simulink model "first_3phase"  (R2015a)
settings: Solver=ode45  StartTime=0.02  StopTime=0.06  RelTol=1e-3
libraries: powerlib x148, powerlib_meascontrol x46, simulink x34
settings Model: Creator=yahya  LastModifiedBy=Yahya

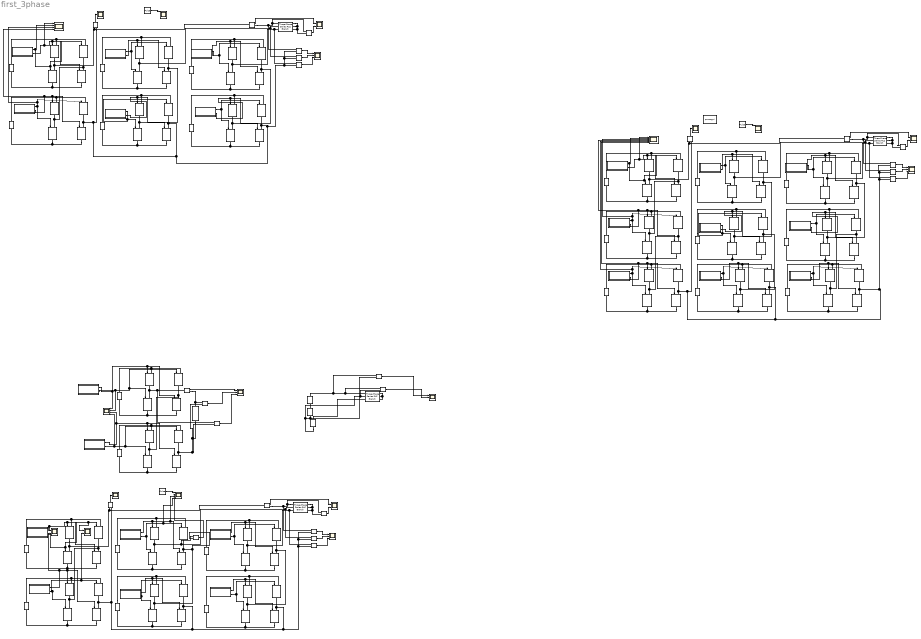
== system first_3phase ==
  note: halate adie swiching
  note: i
  note: i
  note: n
  note: i
  note: n
  note: i
  AC Voltage Source : powerlib/Electrical Sources/AC Voltage Source  Amplitude=100  Phase=0  Frequency=50  SampleTime=0  Measurements=None
  AC Voltage Source1 : powerlib/Electrical Sources/AC Voltage Source  Amplitude=100  Phase=120  Frequency=50  SampleTime=0  Measurements=None
  AC Voltage Source2 : powerlib/Electrical Sources/AC Voltage Source  Amplitude=100  Phase=120  Frequency=50  SampleTime=0  Measurements=None
  Current Measurement{1..4} (4 alike) : powerlib/Measurements/Current Measurement  PhasorSimulation=off  OutputType=Complex  PSBequivalent=0
  DC Voltage Source{1..14,18..26} (23 alike) : powerlib/Electrical Sources/DC Voltage Source  Amplitude=100  Measurements=None
  IGBT/Diode{1..56,69..104} (92 alike) : powerlib/Power Electronics/IGBT//Diode  Ron=1e-3  Rs=1e5  Cs=inf  Measurements=off
  Pulse Generator1 : DiscretePulseGenerator  PulseType=Time based  Amplitude=0.8  Period=0.0001  PulseWidth=50
  Pulse Generator2 : DiscretePulseGenerator  PulseType=Time based  Amplitude=0.8  Period=0.0002  PulseWidth=50
  Pulse Generator3 : DiscretePulseGenerator  PulseType=Time based  Amplitude=0.8  Period=0.0001  PulseWidth=50
  Scope{1,3,6,9,11} (5 alike) : Scope  NumInputPorts=4
      Scope1 settings: YMin=-5~-5~-5~-5  YMax=5~5~5~5
      Scope11 settings: YMin=-5~-5~-5~-5  YMax=5~5~5~5  SaveName=ScopeData10
      Scope3 settings: YMin=-5~-5~-5~-5  YMax=5~5~5~5  SaveName=ScopeData2
      Scope6 settings: YMin=-5~-5~-5~-5  YMax=5~5~5~5  SaveName=ScopeData12
      Scope9 settings: YMin=-5~-5~-5~-5  YMax=5~5~5~5  SaveName=ScopeData18
  Scope{2,5,10,15,17} (5 alike) : Scope  NumInputPorts=3
      Scope10 settings: YMin=-5~-5~-5  YMax=5~5~5  SaveName=ScopeData4
      Scope15 settings: TimeRange=1  YMin=-400~-400~-5  YMax=400~400~5  SaveName=ScopeData14
      Scope17 settings: YMin=-5~-5~-5  YMax=5~5~5  SaveName=ScopeData15
      Scope2 settings: YMin=-5~-5~-5  YMax=5~5~5
      Scope5 settings: TimeRange=1  YMin=-200~-200~-1  YMax=200~200~1  SaveName=ScopeData3
  Scope{4,7,12,14,18} (5 alike) : Scope  NumInputPorts=2
      Scope12 settings: TimeRange=1  YMin=-400~-400  YMax=400~400  SaveName=ScopeData5
      Scope14 settings: YMin=-5~-5  YMax=5~5  SaveName=ScopeData11
      Scope18 settings: TimeRange=1  YMin=-400~-400  YMax=400~400  SaveName=ScopeData16
      Scope4 settings: TimeRange=1  YMin=-400~-400  YMax=400~400  SaveName=ScopeData6
      Scope7 settings: YMin=-5~-5  YMax=5~5  SaveName=ScopeData13
  Scope13 : Scope
      settings: SaveName=ScopeData9
  Scope16 : Scope  NumInputPorts=6
      settings: YMin=-5~-5~-5~-5~-5~-5  YMax=5~5~5~5~5~5  SaveName=ScopeData8
  Scope19 : Scope
      settings: SaveName=ScopeData17
  Scope8 : Scope
      settings: SaveName=ScopeData7
  Series RLC Branch5 : powerlib/Elements/Series RLC Branch  LConnTagsString=__new0  RConnTagsString=__new0  BranchType=R  Resistance=1  Inductance=1e-5  SetiL0=off  InitialCurrent=0  Capacitance=1e-6  Setx0=off  InitialVoltage=0  Measurements=None
  Three-Phase Series RLC Branch : powerlib/Elements/Three-Phase Series RLC Branch  LConnTagsString=A|B|C  RConnTagsString=A|B|C  BranchType=RL  Resistance=1.405*2  Inductance=0.005839*2  Capacitance=1e-6  Measurements=Branch voltages
  Three-Phase Series RLC Branch1 : powerlib/Elements/Three-Phase Series RLC Branch  LConnTagsString=A|B|C  RConnTagsString=A|B|C  BranchType=R  Resistance=1  Inductance=1e-3  Capacitance=1e-6  Measurements=None
  Three-Phase Series RLC Branch2 : powerlib/Elements/Three-Phase Series RLC Branch  LConnTagsString=A|B|C  RConnTagsString=A|B|C  BranchType=R  Resistance=1  Inductance=1e-3  Capacitance=1e-6  Measurements=None
  Three-Phase Series RLC Branch3 : powerlib/Elements/Three-Phase Series RLC Branch  LConnTagsString=A|B|C  RConnTagsString=A|B|C  BranchType=RL  Resistance=1.405*2  Inductance=0.005839*2  Capacitance=1e-6  Measurements=Branch voltages
  Voltage Measurement{1..19} (19 alike) : powerlib/Measurements/Voltage Measurement  PhasorSimulation=off  OutputType=Complex  PSBequivalent=0
  Voltage phase n2 : powerlib/Measurements/Voltage Measurement  PhasorSimulation=off  OutputType=Complex  PSBequivalent=0
  position controller : Subsystem
  position controller1 : Subsystem
  position controller10 : Subsystem
  position controller11 : Subsystem
  position controller12 : Subsystem
  position controller13 : Subsystem
  position controller17 : Subsystem
  position controller18 : Subsystem
  position controller19 : Subsystem
  position controller2 : Subsystem
  position controller20 : Subsystem
  position controller21 : Subsystem
  position controller22 : Subsystem
  position controller23 : Subsystem
  position controller24 : Subsystem
  position controller25 : Subsystem
  position controller3 : Subsystem
  position controller4 : Subsystem
  position controller5 : Subsystem
  position controller6 : Subsystem
  position controller7 : Subsystem
  position controller8 : Subsystem
  position controller9 : Subsystem
  powergui : powerlib/powergui  Priority=1  SimulationMode=Continuous  SolverType=Tustin/Backward Euler (TBE)  SampleTime=50e-6  frequency=60  SPID=off  DisableSnubberDevices=off  DisableRonSwitches=off  DisableVfSwitches=off  SwTol=0  DisplayEquations=off  Interpol=off  methode=off  Ts=100  FunctionMessages=off  echomessages=off  HookPort=off  EnableUseOfTLC=off  x0status=blocks  frequencyindice=0  Pbase=100e6  ErrMax=1e-4  Iterations=50  UnitsV=kV  UnitsW=MW  buscounter=0  RestoreLinks=warning  ResistiveCurrentMeasurement=off  Frange=[0:2:500]  Ylog=off  Xlog=on  ShowGrid=off  save=off  variable=ZData  structure=0  ZoomFFT=on  StartTime=0.0  cycles=1  DisplayStyle=1  fundamental=60  FreqAxis=off  MaxFrequency=1000  frequencyindicesteady=1  RmsSteady=1  display=off
  wires:
  position controller/2(Out2) -> Scope11/1, IGBT/Diode35/1, IGBT/Diode21/1
  Pulse Generator1/1 -> Scope1/1
  Current Measurement2/1 -> Scope4/1
  position controller/1(Out1) -> Scope11/2, IGBT/Diode34/1, IGBT/Diode32/1
  position controller1/2(Out2) -> Scope11/4, IGBT/Diode4/1, IGBT/Diode1/1
  position controller1/1(Out1) -> IGBT/Diode3/1, Scope11/3, IGBT/Diode2/1
  position controller4/2(Out2) -> IGBT/Diode11/1, IGBT/Diode7/1
  position controller4/1(Out1) -> IGBT/Diode10/1, IGBT/Diode9/1
  position controller5/2(Out2) -> IGBT/Diode12/1, IGBT/Diode5/1
  position controller5/1(Out1) -> IGBT/Diode8/1, IGBT/Diode6/1
  position controller6/2(Out2) -> IGBT/Diode14/1, IGBT/Diode18/1
  position controller6/1(Out1) -> IGBT/Diode20/1, IGBT/Diode13/1
  position controller7/2(Out2) -> IGBT/Diode15/1, IGBT/Diode16/1
  position controller7/1(Out1) -> IGBT/Diode19/1, IGBT/Diode17/1
  position controller2/1(Out3) -> IGBT/Diode28/1, IGBT/Diode24/1, Scope3/1
  position controller2/2(Out4) -> Scope3/2, IGBT/Diode26/1, IGBT/Diode27/1
  position controller3/1(Out3) -> Scope3/3, IGBT/Diode29/1, IGBT/Diode22/1
  position controller3/2(Out4) -> Scope3/4, IGBT/Diode25/1, IGBT/Diode23/1
  Current Measurement1/1 -> Scope5/1
  Voltage Measurement5/1 -> Scope5/2
  Voltage Measurement7/1 -> Scope8/1
  Voltage Measurement4/1 -> Scope5/3
  Voltage Measurement1/1 -> Scope4/2
  Voltage Measurement2/1 -> Scope2/1
  Voltage Measurement3/1 -> Scope2/2
  Voltage Measurement6/1 -> Scope2/3
  position controller8/1(Out1) -> Scope14/1, IGBT/Diode50/1, IGBT/Diode46/1
  Current Measurement3/1 -> Scope12/1
  position controller8/2(Out2) -> IGBT/Diode49/1, Scope7/1, IGBT/Diode48/1
  position controller9/1(Out1) -> Scope14/2, IGBT/Diode51/1, IGBT/Diode30/1
  position controller9/2(Out2) -> IGBT/Diode47/1, IGBT/Diode44/1, Scope7/2
  position controller10/1(Out1) -> Scope6/3, IGBT/Diode33/1, IGBT/Diode54/1
  position controller10/2(Out2) -> Scope6/4, IGBT/Diode56/1, IGBT/Diode31/1
  position controller11/1(Out1) -> IGBT/Diode36/1, IGBT/Diode52/1
  position controller11/2(Out2) -> IGBT/Diode55/1, IGBT/Diode53/1
  position controller12/1(Out1) -> IGBT/Diode38/1, IGBT/Diode42/1
  position controller12/2(Out2) -> IGBT/Diode45/1, IGBT/Diode37/1
  position controller13/1(Out1) -> IGBT/Diode39/1, IGBT/Diode40/1
  position controller13/2(Out2) -> IGBT/Diode41/1, IGBT/Diode43/1
  Voltage phase n2/1 -> Scope13/1
  Voltage Measurement8/1 -> Scope12/2
  Voltage Measurement9/1 -> Scope10/1
  Voltage Measurement10/1 -> Scope10/2
  Voltage Measurement11/1 -> Scope10/3
  Voltage Measurement12/1 -> Scope6/2
  Pulse Generator2/1 -> Scope6/1
  Voltage Measurement14/1 -> Scope15/2
  Voltage Measurement13/1 -> Scope15/1
  position controller17/2(Out2) -> Scope16/1, IGBT/Diode86/1, IGBT/Diode82/1
  Pulse Generator3/1 -> Scope9/1
  Current Measurement4/1 -> Scope18/1
  position controller17/1(Out1) -> Scope16/2, IGBT/Diode85/1, IGBT/Diode84/1
  position controller18/2(Out2) -> Scope16/4, IGBT/Diode87/1, IGBT/Diode69/1
  position controller18/1(Out1) -> IGBT/Diode83/1, Scope16/3, IGBT/Diode80/1
  position controller22/2(Out2) -> IGBT/Diode71/1, IGBT/Diode102/1
  position controller22/1(Out1) -> IGBT/Diode70/1, IGBT/Diode104/1
  position controller23/2(Out2) -> IGBT/Diode72/1, IGBT/Diode88/1
  position controller23/1(Out1) -> IGBT/Diode103/1, IGBT/Diode92/1
  position controller24/2(Out2) -> IGBT/Diode74/1, IGBT/Diode78/1
  position controller24/1(Out1) -> IGBT/Diode81/1, IGBT/Diode73/1
  position controller25/2(Out2) -> IGBT/Diode75/1, IGBT/Diode76/1
  position controller25/1(Out1) -> IGBT/Diode79/1, IGBT/Diode77/1
  Voltage Measurement19/1 -> Scope19/1
  Voltage Measurement15/1 -> Scope18/2
  Voltage Measurement16/1 -> Scope17/1
  Voltage Measurement17/1 -> Scope17/2
  Voltage Measurement18/1 -> Scope17/3
  position controller19/2(Out2) -> Scope16/6, IGBT/Diode93/1, IGBT/Diode89/1
  position controller19/1(Out1) -> IGBT/Diode91/1, Scope16/5, IGBT/Diode90/1
  position controller20/2(Out2) -> IGBT/Diode97/1, IGBT/Diode94/1
  position controller20/1(Out1) -> IGBT/Diode96/1, IGBT/Diode95/1
  position controller21/2(Out2) -> IGBT/Diode101/1, IGBT/Diode98/1
  position controller21/1(Out1) -> IGBT/Diode100/1, IGBT/Diode99/1
  connections:
  IGBT/Diode21/LConn1 -- DC Voltage Source5/RConn1 -- IGBT/Diode32/LConn1
  IGBT/Diode35/RConn1 -- DC Voltage Source5/LConn1 -- IGBT/Diode34/RConn1
  IGBT/Diode3/LConn1 -- IGBT/Diode35/LConn1 -- IGBT/Diode32/RConn1 -- IGBT/Diode1/RConn1
  IGBT/Diode1/LConn1 -- DC Voltage Source1/RConn1 -- IGBT/Diode2/LConn1
  IGBT/Diode3/RConn1 -- DC Voltage Source1/LConn1 -- IGBT/Diode4/RConn1
  IGBT/Diode7/LConn1 -- DC Voltage Source3/RConn1 -- IGBT/Diode9/LConn1
  IGBT/Diode10/RConn1 -- DC Voltage Source3/LConn1 -- IGBT/Diode11/RConn1
  IGBT/Diode10/LConn1 -- Three-Phase Series RLC Branch/LConn2 -- Voltage Measurement3/LConn1 -- IGBT/Diode7/RConn1
  IGBT/Diode5/LConn1 -- IGBT/Diode6/LConn1 -- DC Voltage Source2/RConn1
  IGBT/Diode8/RConn1 -- DC Voltage Source2/LConn1 -- IGBT/Diode12/RConn1
  IGBT/Diode9/RConn1 -- IGBT/Diode8/LConn1 -- IGBT/Diode5/RConn1 -- IGBT/Diode11/LConn1
  IGBT/Diode18/LConn1 -- DC Voltage Source6/RConn1 -- IGBT/Diode20/LConn1
  IGBT/Diode13/RConn1 -- DC Voltage Source6/LConn1 -- IGBT/Diode14/RConn1
  IGBT/Diode16/LConn1 -- DC Voltage Source4/RConn1 -- IGBT/Diode17/LConn1
  IGBT/Diode19/RConn1 -- DC Voltage Source4/LConn1 -- IGBT/Diode15/RConn1
  IGBT/Diode20/RConn1 -- IGBT/Diode14/LConn1 -- IGBT/Diode19/LConn1 -- IGBT/Diode16/RConn1
  IGBT/Diode13/LConn1 -- Three-Phase Series RLC Branch/LConn3 -- Voltage Measurement6/LConn1 -- IGBT/Diode18/RConn1
  IGBT/Diode26/LConn1 -- IGBT/Diode24/LConn1 -- DC Voltage Source8/RConn1
  IGBT/Diode27/RConn1 -- IGBT/Diode28/RConn1 -- DC Voltage Source8/LConn1
  IGBT/Diode27/LConn1 -- Current Measurement1/LConn1 -- Voltage Measurement4/LConn1 -- IGBT/Diode24/RConn1
  IGBT/Diode23/LConn1 -- IGBT/Diode22/LConn1 -- DC Voltage Source7/RConn1
  IGBT/Diode29/RConn1 -- IGBT/Diode25/RConn1 -- DC Voltage Source7/LConn1
  IGBT/Diode28/LConn1 -- IGBT/Diode26/RConn1 -- IGBT/Diode25/LConn1 -- IGBT/Diode22/RConn1
  Series RLC Branch5/LConn1 -- Current Measurement1/RConn1 -- Voltage Measurement5/LConn1
  IGBT/Diode34/LConn1 -- IGBT/Diode21/RConn1 -- Voltage Measurement7/LConn1 -- Current Measurement2/LConn1
  Current Measurement2/RConn1 -- Voltage Measurement1/LConn1 -- Three-Phase Series RLC Branch/LConn1 -- Voltage Measurement2/LConn1
  Voltage Measurement1/LConn2 -- Three-Phase Series RLC Branch/RConn2 -- Three-Phase Series RLC Branch/RConn1 -- Three-Phase Series RLC Branch/RConn3
  IGBT/Diode48/LConn1 -- IGBT/Diode46/LConn1 -- DC Voltage Source13/RConn1
  IGBT/Diode49/RConn1 -- IGBT/Diode50/RConn1 -- DC Voltage Source13/LConn1
  IGBT/Diode30/RConn1 -- IGBT/Diode47/LConn1 -- IGBT/Diode50/LConn1 -- IGBT/Diode48/RConn1
  IGBT/Diode44/LConn1 -- IGBT/Diode30/LConn1 -- DC Voltage Source9/RConn1
  IGBT/Diode51/RConn1 -- IGBT/Diode47/RConn1 -- DC Voltage Source9/LConn1
  IGBT/Diode56/LConn1 -- IGBT/Diode54/LConn1 -- DC Voltage Source11/RConn1
  IGBT/Diode33/RConn1 -- IGBT/Diode31/RConn1 -- DC Voltage Source11/LConn1
  IGBT/Diode54/RConn1 -- Three-Phase Series RLC Branch1/LConn2 -- Voltage Measurement10/LConn1 -- Voltage Measurement12/LConn1 -- IGBT/Diode31/LConn1
  DC Voltage Source10/RConn1 -- IGBT/Diode52/LConn1 -- IGBT/Diode53/LConn1
  IGBT/Diode36/RConn1 -- IGBT/Diode55/RConn1 -- DC Voltage Source10/LConn1
  IGBT/Diode33/LConn1 -- IGBT/Diode56/RConn1 -- IGBT/Diode55/LConn1 -- IGBT/Diode52/RConn1 -- Voltage Measurement12/LConn2
  IGBT/Diode45/LConn1 -- DC Voltage Source14/RConn1 -- IGBT/Diode42/LConn1
  IGBT/Diode38/RConn1 -- IGBT/Diode37/RConn1 -- DC Voltage Source14/LConn1
  IGBT/Diode41/LConn1 -- DC Voltage Source12/RConn1 -- IGBT/Diode40/LConn1
  IGBT/Diode39/RConn1 -- IGBT/Diode43/RConn1 -- DC Voltage Source12/LConn1
  IGBT/Diode40/RConn1 -- IGBT/Diode43/LConn1 -- IGBT/Diode45/RConn1 -- IGBT/Diode38/LConn1
  IGBT/Diode42/RConn1 -- Three-Phase Series RLC Branch1/LConn3 -- Voltage Measurement11/LConn1 -- IGBT/Diode37/LConn1
  Voltage phase n2/LConn1 -- Current Measurement3/LConn1 -- IGBT/Diode49/LConn1 -- IGBT/Diode46/RConn1
  Three-Phase Series RLC Branch1/LConn1 -- Voltage Measurement9/LConn1 -- Current Measurement3/RConn1 -- Voltage Measurement8/LConn1
  Three-Phase Series RLC Branch1/RConn1 -- Voltage Measurement8/LConn2 -- Three-Phase Series RLC Branch1/RConn3 -- Three-Phase Series RLC Branch1/RConn2
  IGBT/Diode53/RConn1 -- IGBT/Diode39/LConn1 -- IGBT/Diode41/RConn1 -- Voltage Measurement11/LConn2 -- Voltage Measurement9/LConn2 -- Voltage Measurement10/LConn2 -- Voltage phase n2/LConn2 -- IGBT/Diode51/LConn1 -- IGBT/Diode44/RConn1 -- IGBT/Diode36/LConn1
  AC Voltage Source1/LConn1 -- AC Voltage Source/LConn1 -- AC Voltage Source2/LConn1 -- Voltage Measurement13/LConn2
  AC Voltage Source/RConn1 -- Voltage Measurement13/LConn1 -- Voltage Measurement14/LConn1 -- Three-Phase Series RLC Branch2/LConn1
  AC Voltage Source1/RConn1 -- Voltage Measurement14/LConn2 -- Three-Phase Series RLC Branch2/LConn2
  AC Voltage Source2/RConn1 -- Three-Phase Series RLC Branch2/LConn3
  Three-Phase Series RLC Branch2/RConn1 -- Three-Phase Series RLC Branch2/RConn3 -- Three-Phase Series RLC Branch2/RConn2
  Voltage Measurement5/LConn2 -- Series RLC Branch5/RConn1 -- IGBT/Diode29/LConn1 -- IGBT/Diode23/RConn1 -- Voltage Measurement4/LConn2
  IGBT/Diode4/LConn1 -- Voltage Measurement6/LConn2 -- Voltage Measurement2/LConn2 -- Voltage Measurement3/LConn2 -- IGBT/Diode17/RConn1 -- IGBT/Diode15/LConn1 -- IGBT/Diode6/RConn1 -- IGBT/Diode12/LConn1 -- Voltage Measurement7/LConn2 -- IGBT/Diode2/RConn1
  IGBT/Diode84/LConn1 -- IGBT/Diode82/LConn1 -- DC Voltage Source25/RConn1
  IGBT/Diode85/RConn1 -- IGBT/Diode86/RConn1 -- DC Voltage Source25/LConn1
  IGBT/Diode69/RConn1 -- IGBT/Diode83/LConn1 -- IGBT/Diode86/LConn1 -- IGBT/Diode84/RConn1
  IGBT/Diode80/LConn1 -- IGBT/Diode69/LConn1 -- DC Voltage Source18/RConn1
  IGBT/Diode87/RConn1 -- IGBT/Diode83/RConn1 -- DC Voltage Source18/LConn1
  IGBT/Diode104/LConn1 -- IGBT/Diode102/LConn1 -- DC Voltage Source23/RConn1
  IGBT/Diode71/RConn1 -- IGBT/Diode70/RConn1 -- DC Voltage Source23/LConn1
  IGBT/Diode102/RConn1 -- IGBT/Diode70/LConn1 -- Three-Phase Series RLC Branch3/LConn2 -- Voltage Measurement17/LConn1
  DC Voltage Source22/RConn1 -- IGBT/Diode88/LConn1 -- IGBT/Diode92/LConn1
  IGBT/Diode72/RConn1 -- IGBT/Diode103/RConn1 -- DC Voltage Source22/LConn1
  IGBT/Diode71/LConn1 -- IGBT/Diode104/RConn1 -- IGBT/Diode103/LConn1 -- IGBT/Diode88/RConn1
  IGBT/Diode81/LConn1 -- IGBT/Diode78/LConn1 -- DC Voltage Source26/RConn1
  IGBT/Diode74/RConn1 -- IGBT/Diode73/RConn1 -- DC Voltage Source26/LConn1
  IGBT/Diode77/LConn1 -- IGBT/Diode76/LConn1 -- DC Voltage Source24/RConn1
  IGBT/Diode75/RConn1 -- IGBT/Diode79/RConn1 -- DC Voltage Source24/LConn1
  IGBT/Diode76/RConn1 -- IGBT/Diode79/LConn1 -- IGBT/Diode81/RConn1 -- IGBT/Diode74/LConn1
  IGBT/Diode78/RConn1 -- Three-Phase Series RLC Branch3/LConn3 -- Voltage Measurement18/LConn1 -- IGBT/Diode73/LConn1
  Current Measurement4/LConn1 -- Voltage Measurement19/LConn1 -- IGBT/Diode85/LConn1 -- IGBT/Diode82/RConn1
  Voltage Measurement16/LConn1 -- Current Measurement4/RConn1 -- Voltage Measurement15/LConn1 -- Three-Phase Series RLC Branch3/LConn1
  Three-Phase Series RLC Branch3/RConn3 -- Voltage Measurement15/LConn2 -- Three-Phase Series RLC Branch3/RConn2 -- Three-Phase Series RLC Branch3/RConn1
  IGBT/Diode91/LConn1 -- IGBT/Diode80/RConn1 -- IGBT/Diode87/LConn1 -- IGBT/Diode89/RConn1
  IGBT/Diode96/LConn1 -- IGBT/Diode92/RConn1 -- IGBT/Diode72/LConn1 -- IGBT/Diode94/RConn1
  IGBT/Diode100/LConn1 -- IGBT/Diode77/RConn1 -- IGBT/Diode75/LConn1 -- IGBT/Diode98/RConn1
  IGBT/Diode90/LConn1 -- IGBT/Diode89/LConn1 -- DC Voltage Source19/RConn1
  IGBT/Diode93/RConn1 -- IGBT/Diode91/RConn1 -- DC Voltage Source19/LConn1
  IGBT/Diode95/LConn1 -- IGBT/Diode94/LConn1 -- DC Voltage Source20/RConn1
  IGBT/Diode97/RConn1 -- IGBT/Diode96/RConn1 -- DC Voltage Source20/LConn1
  IGBT/Diode99/LConn1 -- IGBT/Diode98/LConn1 -- DC Voltage Source21/RConn1
  IGBT/Diode101/RConn1 -- IGBT/Diode100/RConn1 -- DC Voltage Source21/LConn1
  IGBT/Diode95/RConn1 -- IGBT/Diode97/LConn1 -- Voltage Measurement16/LConn2 -- Voltage Measurement17/LConn2 -- Voltage Measurement18/LConn2 -- IGBT/Diode99/RConn1 -- IGBT/Diode101/LConn1 -- Voltage Measurement19/LConn2 -- IGBT/Diode90/RConn1 -- IGBT/Diode93/LConn1

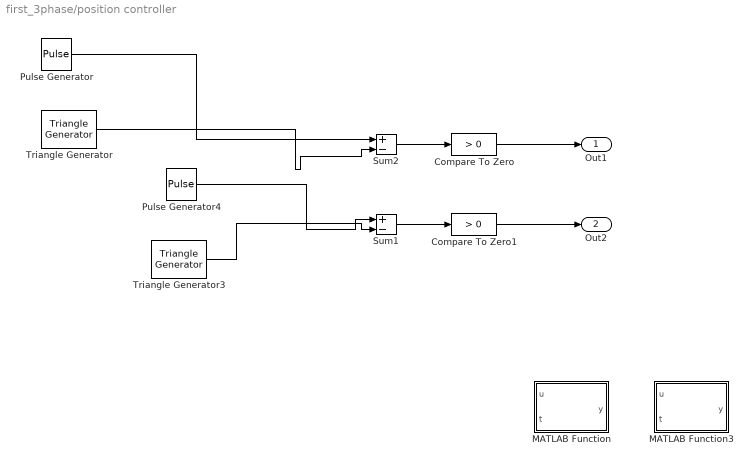
== system first_3phase/position controller ==
  Compare To Zero : simulink/Logic and Bit Operations/Compare To Zero  relop=>  OutDataTypeStr=boolean  ZeroCross=off
  Compare To Zero1 : simulink/Logic and Bit Operations/Compare To Zero  relop=>  OutDataTypeStr=boolean  ZeroCross=off
  MATLAB Function : MATLAB Function  TreatAsAtomicUnit=on
  MATLAB Function3 : MATLAB Function  TreatAsAtomicUnit=on
  Pulse Generator : DiscretePulseGenerator  PulseType=Time based  Amplitude=0.666  Period=0.02  PulseWidth=50
  Pulse Generator4 : DiscretePulseGenerator  PulseType=Time based  Amplitude=0.666  Period=0.02  PulseWidth=50  PhaseDelay=0.01
  Sum1 : Sum  Inputs=+-  OutDataTypeStr=double
  Sum2 : Sum  Inputs=+-  OutDataTypeStr=double
  Triangle Generator : powerlib_meascontrol/Pulse & Signal Generators/Triangle Generator  Freq=50  Phase=90  Ts=0
  Triangle Generator3 : powerlib_meascontrol/Pulse & Signal Generators/Triangle Generator  Freq=50  Phase=90+180  Ts=0
  Out1 : Outport
  Out2 : Outport  Port=2
  wires:
  Compare To Zero/1 -> Out1/1
  Pulse Generator/1 -> Sum2/1
  Triangle Generator/1 -> Sum2/2
  Pulse Generator4/1 -> Sum1/1
  Triangle Generator3/1 -> Sum1/2
  Compare To Zero1/1 -> Out2/1
  Sum2/1 -> Compare To Zero/1
  Sum1/1 -> Compare To Zero1/1

== system first_3phase/position controller1 ==
  Compare To Zero : simulink/Logic and Bit Operations/Compare To Zero  relop=>  OutDataTypeStr=boolean  ZeroCross=off
  Compare To Zero1 : simulink/Logic and Bit Operations/Compare To Zero  relop=>  OutDataTypeStr=boolean  ZeroCross=off
  Pulse Generator5 : DiscretePulseGenerator  PulseType=Time based  Amplitude=0.333  Period=0.02  PulseWidth=50
  Pulse Generator6 : DiscretePulseGenerator  PulseType=Time based  Amplitude=0.333  Period=0.02  PulseWidth=50  PhaseDelay=0.01
  Sum1 : Sum  Inputs=+-  OutDataTypeStr=double
  Sum2 : Sum  Inputs=+-  OutDataTypeStr=double
  Triangle Generator4 : powerlib_meascontrol/Pulse & Signal Generators/Triangle Generator  Freq=50  Phase=90  Ts=0
  Triangle Generator5 : powerlib_meascontrol/Pulse & Signal Generators/Triangle Generator  Freq=50  Phase=90+180  Ts=0
  Out1 : Outport
  Out2 : Outport  Port=2
  wires:
  Compare To Zero/1 -> Out1/1
  Compare To Zero1/1 -> Out2/1
  Pulse Generator5/1 -> Sum2/1
  Triangle Generator4/1 -> Sum2/2
  Pulse Generator6/1 -> Sum1/1
  Triangle Generator5/1 -> Sum1/2
  Sum2/1 -> Compare To Zero/1
  Sum1/1 -> Compare To Zero1/1

== system first_3phase/position controller10 ==
  Clock : Clock
  Pulse Generator7 : DiscretePulseGenerator  PulseType=Time based  Period=0.02  PulseWidth=50  PhaseDelay=0.00666
  Pulse Generator8 : DiscretePulseGenerator  PulseType=Time based  Period=0.02  PulseWidth=50  PhaseDelay=0.01+0.00666
  Triangle Generator6 : powerlib_meascontrol/Pulse & Signal Generators/Triangle Generator  Freq=50  Phase=90+240  Ts=0
  Triangle Generator7 : powerlib_meascontrol/Pulse & Signal Generators/Triangle Generator  Freq=50  Phase=90+180+240  Ts=0
  Out1 : Outport
  Out2 : Outport  Port=2
  wires:
  Pulse Generator7/1 -> Out1/1
  Pulse Generator8/1 -> Out2/1
  Triangle Generator6/1 -> ?
  Triangle Generator7/1 -> ?
  Clock/1 -> ?

== system first_3phase/position controller11 ==
  Clock : Clock
  MATLAB Function8 : MATLAB Function  TreatAsAtomicUnit=on
  MATLAB Function9 : MATLAB Function  TreatAsAtomicUnit=on
  Pulse Generator10 : DiscretePulseGenerator  PulseType=Time based  Amplitude=0.332  Period=0.02  PulseWidth=50  PhaseDelay=0.01+0.00666
  Pulse Generator9 : DiscretePulseGenerator  PulseType=Time based  Amplitude=0.332  Period=0.02  PulseWidth=50  PhaseDelay=0.00666
  Triangle Generator8 : powerlib_meascontrol/Pulse & Signal Generators/Triangle Generator  Freq=50  Phase=90+240  Ts=0
  Triangle Generator9 : powerlib_meascontrol/Pulse & Signal Generators/Triangle Generator  Freq=50  Phase=90+180+240  Ts=0
  Out1 : Outport
  Out2 : Outport  Port=2
  wires:
  MATLAB Function8/1(y) -> Out1/1
  Pulse Generator9/1 -> MATLAB Function8/1(u)
  Triangle Generator8/1 -> MATLAB Function8/2(t)
  MATLAB Function9/1(y) -> Out2/1
  Pulse Generator10/1 -> MATLAB Function9/1(u)
  Triangle Generator9/1 -> MATLAB Function9/3(t)
  Clock/1 -> MATLAB Function9/2(c)

== system first_3phase/position controller12 ==
  Clock : Clock
  Pulse Generator12 : DiscretePulseGenerator  PulseType=Time based  Period=0.02  PulseWidth=50  PhaseDelay=0.00666*2
  Pulse Generator13 : DiscretePulseGenerator  PulseType=Time based  Period=0.02  PulseWidth=50  PhaseDelay=0.01+0.00666*2
  Triangle Generator10 : powerlib_meascontrol/Pulse & Signal Generators/Triangle Generator  Freq=50  Phase=90+120  Ts=0
  Triangle Generator11 : powerlib_meascontrol/Pulse & Signal Generators/Triangle Generator  Freq=50  Phase=90+180+120  Ts=0
  Out1 : Outport
  Out2 : Outport  Port=2
  wires:
  Pulse Generator12/1 -> Out1/1
  Pulse Generator13/1 -> Out2/1
  Triangle Generator10/1 -> ?
  Triangle Generator11/1 -> ?
  Clock/1 -> ?

== system first_3phase/position controller13 ==
  Clock : Clock
  Pulse Generator11 : DiscretePulseGenerator  PulseType=Time based  Period=0.02  PulseWidth=50  PhaseDelay=0.01+0.00666*2
  Pulse Generator14 : DiscretePulseGenerator  PulseType=Time based  Amplitude=2  Period=0.02  PulseWidth=50  PhaseDelay=0.00666*2
  Triangle Generator12 : powerlib_meascontrol/Pulse & Signal Generators/Triangle Generator  Freq=50  Phase=90+120  Ts=0
  Triangle Generator13 : powerlib_meascontrol/Pulse & Signal Generators/Triangle Generator  Freq=50  Phase=90+180+120  Ts=0
  Out1 : Outport
  Out2 : Outport  Port=2
  wires:
  Pulse Generator14/1 -> Out1/1
  Pulse Generator11/1 -> Out2/1
  Triangle Generator12/1 -> ?
  Triangle Generator13/1 -> ?
  Clock/1 -> ?

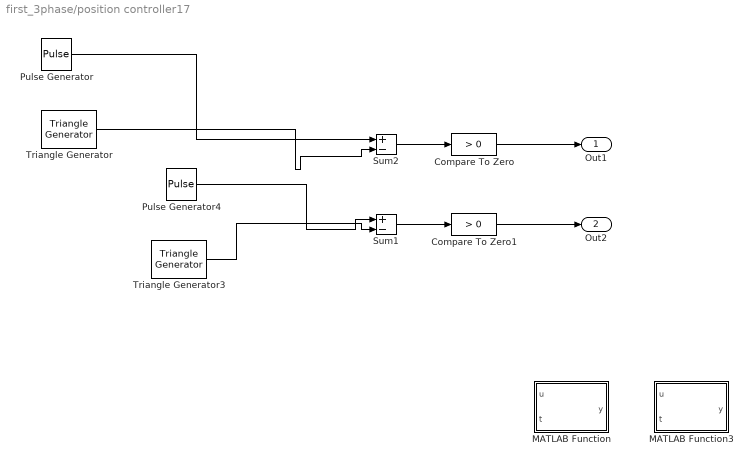
== system first_3phase/position controller17 ==
  Compare To Zero : simulink/Logic and Bit Operations/Compare To Zero  relop=>  OutDataTypeStr=boolean  ZeroCross=off
  Compare To Zero1 : simulink/Logic and Bit Operations/Compare To Zero  relop=>  OutDataTypeStr=boolean  ZeroCross=off
  MATLAB Function : MATLAB Function  TreatAsAtomicUnit=on
  MATLAB Function3 : MATLAB Function  TreatAsAtomicUnit=on
  Pulse Generator : DiscretePulseGenerator  PulseType=Time based  Amplitude=0.9774  Period=0.02  PulseWidth=50
  Pulse Generator4 : DiscretePulseGenerator  PulseType=Time based  Amplitude=0.9774  Period=0.02  PulseWidth=50  PhaseDelay=0.01
  Sum1 : Sum  Inputs=+-  OutDataTypeStr=double
  Sum2 : Sum  Inputs=+-  OutDataTypeStr=double
  Triangle Generator : powerlib_meascontrol/Pulse & Signal Generators/Triangle Generator  Freq=50  Phase=90  Ts=0
  Triangle Generator3 : powerlib_meascontrol/Pulse & Signal Generators/Triangle Generator  Freq=50  Phase=90+180  Ts=0
  Out1 : Outport
  Out2 : Outport  Port=2
  wires:
  Compare To Zero/1 -> Out1/1
  Pulse Generator/1 -> Sum2/1
  Triangle Generator/1 -> Sum2/2
  Pulse Generator4/1 -> Sum1/1
  Triangle Generator3/1 -> Sum1/2
  Compare To Zero1/1 -> Out2/1
  Sum2/1 -> Compare To Zero/1
  Sum1/1 -> Compare To Zero1/1

== system first_3phase/position controller18 ==
  Compare To Zero : simulink/Logic and Bit Operations/Compare To Zero  relop=>  OutDataTypeStr=boolean  ZeroCross=off
  Compare To Zero1 : simulink/Logic and Bit Operations/Compare To Zero  relop=>  OutDataTypeStr=boolean  ZeroCross=off
  Pulse Generator5 : DiscretePulseGenerator  PulseType=Time based  Amplitude=0.9502  Period=0.02  PulseWidth=50
  Pulse Generator6 : DiscretePulseGenerator  PulseType=Time based  Amplitude=0.9502  Period=0.02  PulseWidth=50  PhaseDelay=0.01
  Sum1 : Sum  Inputs=+-  OutDataTypeStr=double
  Sum2 : Sum  Inputs=+-  OutDataTypeStr=double
  Triangle Generator4 : powerlib_meascontrol/Pulse & Signal Generators/Triangle Generator  Freq=50  Phase=90  Ts=0
  Triangle Generator5 : powerlib_meascontrol/Pulse & Signal Generators/Triangle Generator  Freq=50  Phase=90+180  Ts=0
  Out1 : Outport
  Out2 : Outport  Port=2
  wires:
  Compare To Zero/1 -> Out1/1
  Compare To Zero1/1 -> Out2/1
  Pulse Generator5/1 -> Sum2/1
  Triangle Generator4/1 -> Sum2/2
  Pulse Generator6/1 -> Sum1/1
  Triangle Generator5/1 -> Sum1/2
  Sum2/1 -> Compare To Zero/1
  Sum1/1 -> Compare To Zero1/1

== system first_3phase/position controller19 ==
  Compare To Zero : simulink/Logic and Bit Operations/Compare To Zero  relop=>  OutDataTypeStr=boolean  ZeroCross=off
  Compare To Zero1 : simulink/Logic and Bit Operations/Compare To Zero  relop=>  OutDataTypeStr=boolean  ZeroCross=off
  Pulse Generator5 : DiscretePulseGenerator  PulseType=Time based  Amplitude=0.5294  Period=0.02  PulseWidth=50
  Pulse Generator6 : DiscretePulseGenerator  PulseType=Time based  Amplitude=0.5294  Period=0.02  PulseWidth=50  PhaseDelay=0.01
  Sum1 : Sum  Inputs=+-  OutDataTypeStr=double
  Sum2 : Sum  Inputs=+-  OutDataTypeStr=double
  Triangle Generator4 : powerlib_meascontrol/Pulse & Signal Generators/Triangle Generator  Freq=50  Phase=90  Ts=0
  Triangle Generator5 : powerlib_meascontrol/Pulse & Signal Generators/Triangle Generator  Freq=50  Phase=90+180  Ts=0
  Out1 : Outport
  Out2 : Outport  Port=2
  wires:
  Compare To Zero/1 -> Out1/1
  Compare To Zero1/1 -> Out2/1
  Pulse Generator5/1 -> Sum2/1
  Triangle Generator4/1 -> Sum2/2
  Pulse Generator6/1 -> Sum1/1
  Triangle Generator5/1 -> Sum1/2
  Sum2/1 -> Compare To Zero/1
  Sum1/1 -> Compare To Zero1/1

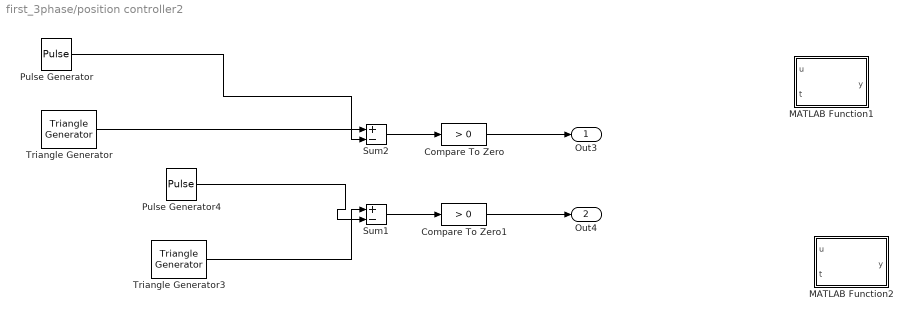
== system first_3phase/position controller2 ==
  Compare To Zero : simulink/Logic and Bit Operations/Compare To Zero  relop=>  OutDataTypeStr=boolean  ZeroCross=off
  Compare To Zero1 : simulink/Logic and Bit Operations/Compare To Zero  relop=>  OutDataTypeStr=boolean  ZeroCross=off
  MATLAB Function1 : MATLAB Function  TreatAsAtomicUnit=on
  MATLAB Function2 : MATLAB Function  TreatAsAtomicUnit=on
  Pulse Generator : DiscretePulseGenerator  PulseType=Time based  Amplitude=0.666  Period=0.02  PulseWidth=50.001
  Pulse Generator4 : DiscretePulseGenerator  PulseType=Time based  Amplitude=0.666  Period=0.02  PulseWidth=50.001  PhaseDelay=0.01
  Sum1 : Sum  Inputs=+-  OutDataTypeStr=double
  Sum2 : Sum  Inputs=+-  OutDataTypeStr=double
  Triangle Generator : powerlib_meascontrol/Pulse & Signal Generators/Triangle Generator  Freq=50  Phase=90  Ts=0
  Triangle Generator3 : powerlib_meascontrol/Pulse & Signal Generators/Triangle Generator  Freq=50  Phase=90+180  Ts=0
  Out3 : Outport
  Out4 : Outport  Port=2
  wires:
  Compare To Zero/1 -> Out3/1
  Pulse Generator/1 -> Sum2/2
  Triangle Generator/1 -> Sum2/1
  Pulse Generator4/1 -> Sum1/2
  Triangle Generator3/1 -> Sum1/1
  Compare To Zero1/1 -> Out4/1
  Sum2/1 -> Compare To Zero/1
  Sum1/1 -> Compare To Zero1/1

== system first_3phase/position controller20 ==
  Compare To Zero : simulink/Logic and Bit Operations/Compare To Zero  relop=>  OutDataTypeStr=boolean  ZeroCross=off
  Compare To Zero1 : simulink/Logic and Bit Operations/Compare To Zero  relop=>  OutDataTypeStr=boolean  ZeroCross=off
  Pulse Generator5 : DiscretePulseGenerator  PulseType=Time based  Amplitude=0.5294  Period=0.02  PulseWidth=50
  Pulse Generator6 : DiscretePulseGenerator  PulseType=Time based  Amplitude=0.5294  Period=0.02  PulseWidth=50  PhaseDelay=0.01
  Sum1 : Sum  Inputs=+-  OutDataTypeStr=double
  Sum2 : Sum  Inputs=+-  OutDataTypeStr=double
  Triangle Generator4 : powerlib_meascontrol/Pulse & Signal Generators/Triangle Generator  Freq=50  Phase=90+240  Ts=0
  Triangle Generator5 : powerlib_meascontrol/Pulse & Signal Generators/Triangle Generator  Freq=50  Phase=90+180+240  Ts=0
  Out1 : Outport
  Out2 : Outport  Port=2
  wires:
  Compare To Zero/1 -> Out1/1
  Compare To Zero1/1 -> Out2/1
  Pulse Generator5/1 -> Sum2/1
  Triangle Generator4/1 -> Sum2/2
  Pulse Generator6/1 -> Sum1/1
  Triangle Generator5/1 -> Sum1/2
  Sum2/1 -> Compare To Zero/1
  Sum1/1 -> Compare To Zero1/1

== system first_3phase/position controller21 ==
  Compare To Zero : simulink/Logic and Bit Operations/Compare To Zero  relop=>  OutDataTypeStr=boolean  ZeroCross=off
  Compare To Zero1 : simulink/Logic and Bit Operations/Compare To Zero  relop=>  OutDataTypeStr=boolean  ZeroCross=off
  Pulse Generator5 : DiscretePulseGenerator  PulseType=Time based  Amplitude=0.5294  Period=0.535476666666667  PulseWidth=50
  Pulse Generator6 : DiscretePulseGenerator  PulseType=Time based  Amplitude=0.5294  Period=0.02  PulseWidth=50  PhaseDelay=0.01
  Sum1 : Sum  Inputs=+-  OutDataTypeStr=double
  Sum2 : Sum  Inputs=+-  OutDataTypeStr=double
  Triangle Generator4 : powerlib_meascontrol/Pulse & Signal Generators/Triangle Generator  Freq=50  Phase=90+120  Ts=0
  Triangle Generator5 : powerlib_meascontrol/Pulse & Signal Generators/Triangle Generator  Freq=50  Phase=90+180+120  Ts=0
  Out1 : Outport
  Out2 : Outport  Port=2
  wires:
  Compare To Zero/1 -> Out1/1
  Compare To Zero1/1 -> Out2/1
  Pulse Generator5/1 -> Sum2/1
  Triangle Generator4/1 -> Sum2/2
  Pulse Generator6/1 -> Sum1/1
  Triangle Generator5/1 -> Sum1/2
  Sum2/1 -> Compare To Zero/1
  Sum1/1 -> Compare To Zero1/1

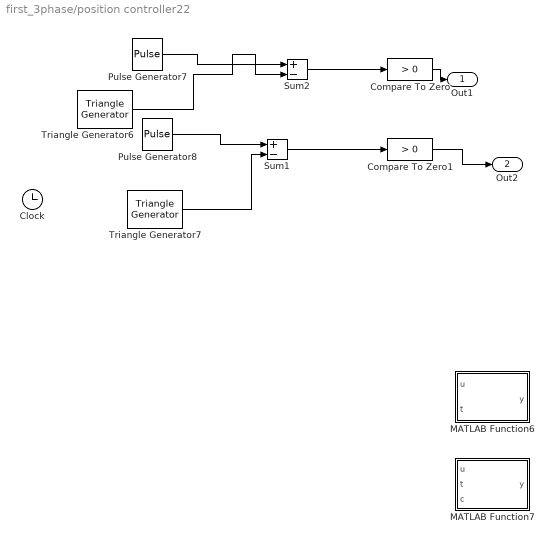
== system first_3phase/position controller22 ==
  Clock : Clock
  Compare To Zero : simulink/Logic and Bit Operations/Compare To Zero  relop=>  OutDataTypeStr=boolean  ZeroCross=off
  Compare To Zero1 : simulink/Logic and Bit Operations/Compare To Zero  relop=>  OutDataTypeStr=boolean  ZeroCross=off
  MATLAB Function6 : MATLAB Function  TreatAsAtomicUnit=on
  MATLAB Function7 : MATLAB Function  TreatAsAtomicUnit=on
  Pulse Generator7 : DiscretePulseGenerator  PulseType=Time based  Amplitude=0.9774  Period=0.02  PulseWidth=50  PhaseDelay=0.00666
  Pulse Generator8 : DiscretePulseGenerator  PulseType=Time based  Amplitude=0.9774  Period=0.02  PulseWidth=50  PhaseDelay=0.01+0.00666
  Sum1 : Sum  Inputs=+-  OutDataTypeStr=double
  Sum2 : Sum  Inputs=+-  OutDataTypeStr=double
  Triangle Generator6 : powerlib_meascontrol/Pulse & Signal Generators/Triangle Generator  Freq=50  Phase=90+240  Ts=0
  Triangle Generator7 : powerlib_meascontrol/Pulse & Signal Generators/Triangle Generator  Freq=50  Phase=90+180+240  Ts=0
  Out1 : Outport
  Out2 : Outport  Port=2
  wires:
  Compare To Zero/1 -> Out1/1
  Compare To Zero1/1 -> Out2/1
  Triangle Generator6/1 -> Sum2/2
  Pulse Generator8/1 -> Sum1/1
  Pulse Generator7/1 -> Sum2/1
  Triangle Generator7/1 -> Sum1/2
  Sum2/1 -> Compare To Zero/1
  Sum1/1 -> Compare To Zero1/1

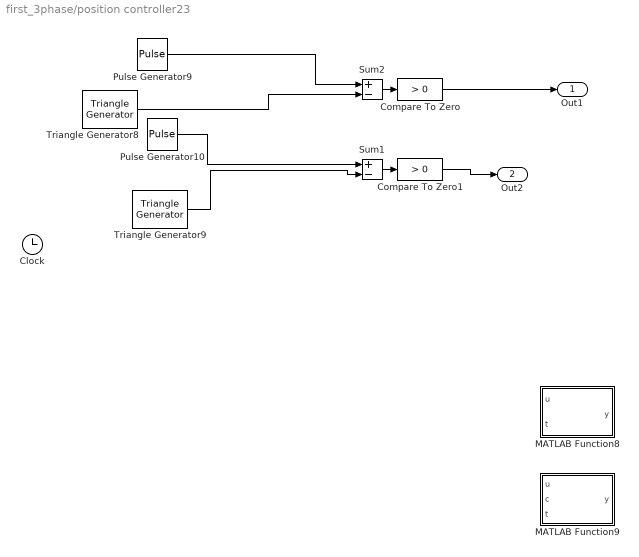
== system first_3phase/position controller23 ==
  Clock : Clock
  Compare To Zero : simulink/Logic and Bit Operations/Compare To Zero  relop=>  OutDataTypeStr=boolean  ZeroCross=off
  Compare To Zero1 : simulink/Logic and Bit Operations/Compare To Zero  relop=>  OutDataTypeStr=boolean  ZeroCross=off
  MATLAB Function8 : MATLAB Function  TreatAsAtomicUnit=on
  MATLAB Function9 : MATLAB Function  TreatAsAtomicUnit=on
  Pulse Generator10 : DiscretePulseGenerator  PulseType=Time based  Amplitude=0.9502  Period=0.02  PulseWidth=50  PhaseDelay=0.01+0.00666
  Pulse Generator9 : DiscretePulseGenerator  PulseType=Time based  Amplitude=0.9502  Period=0.02  PulseWidth=50  PhaseDelay=0.00666
  Sum1 : Sum  Inputs=+-  OutDataTypeStr=double
  Sum2 : Sum  Inputs=+-  OutDataTypeStr=double
  Triangle Generator8 : powerlib_meascontrol/Pulse & Signal Generators/Triangle Generator  Freq=50  Phase=90+240  Ts=0
  Triangle Generator9 : powerlib_meascontrol/Pulse & Signal Generators/Triangle Generator  Freq=50  Phase=90+180+240  Ts=0
  Out1 : Outport
  Out2 : Outport  Port=2
  wires:
  Compare To Zero/1 -> Out1/1
  Triangle Generator8/1 -> Sum2/2
  Compare To Zero1/1 -> Out2/1
  Pulse Generator10/1 -> Sum1/1
  Triangle Generator9/1 -> Sum1/2
  Sum2/1 -> Compare To Zero/1
  Sum1/1 -> Compare To Zero1/1
  Pulse Generator9/1 -> Sum2/1

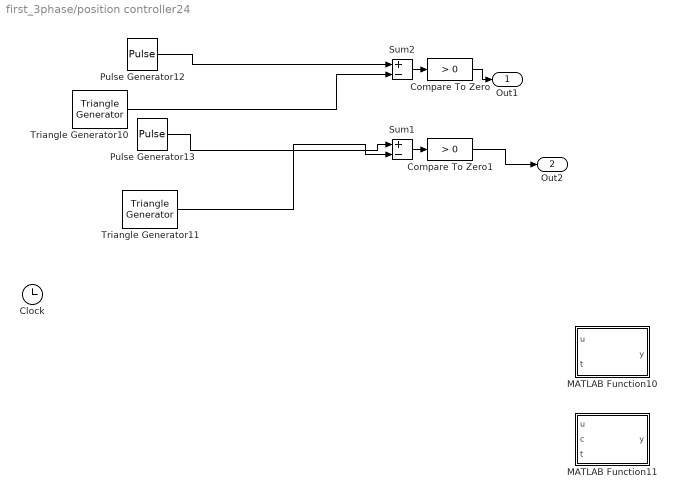
== system first_3phase/position controller24 ==
  Clock : Clock
  Compare To Zero : simulink/Logic and Bit Operations/Compare To Zero  relop=>  OutDataTypeStr=boolean  ZeroCross=off
  Compare To Zero1 : simulink/Logic and Bit Operations/Compare To Zero  relop=>  OutDataTypeStr=boolean  ZeroCross=off
  MATLAB Function10 : MATLAB Function  TreatAsAtomicUnit=on
  MATLAB Function11 : MATLAB Function  TreatAsAtomicUnit=on
  Pulse Generator12 : DiscretePulseGenerator  PulseType=Time based  Amplitude=0.9774  Period=0.02  PulseWidth=50  PhaseDelay=0.00666*2
  Pulse Generator13 : DiscretePulseGenerator  PulseType=Time based  Amplitude=0.9774  Period=0.02  PulseWidth=50  PhaseDelay=0.01+0.00666*2
  Sum1 : Sum  Inputs=+-  OutDataTypeStr=double
  Sum2 : Sum  Inputs=+-  OutDataTypeStr=double
  Triangle Generator10 : powerlib_meascontrol/Pulse & Signal Generators/Triangle Generator  Freq=50  Phase=90+120  Ts=0
  Triangle Generator11 : powerlib_meascontrol/Pulse & Signal Generators/Triangle Generator  Freq=50  Phase=90+180+120  Ts=0
  Out1 : Outport
  Out2 : Outport  Port=2
  wires:
  Compare To Zero/1 -> Out1/1
  Compare To Zero1/1 -> Out2/1
  Triangle Generator10/1 -> Sum2/2
  Pulse Generator13/1 -> Sum1/1
  Triangle Generator11/1 -> Sum1/2
  Pulse Generator12/1 -> Sum2/1
  Sum2/1 -> Compare To Zero/1
  Sum1/1 -> Compare To Zero1/1

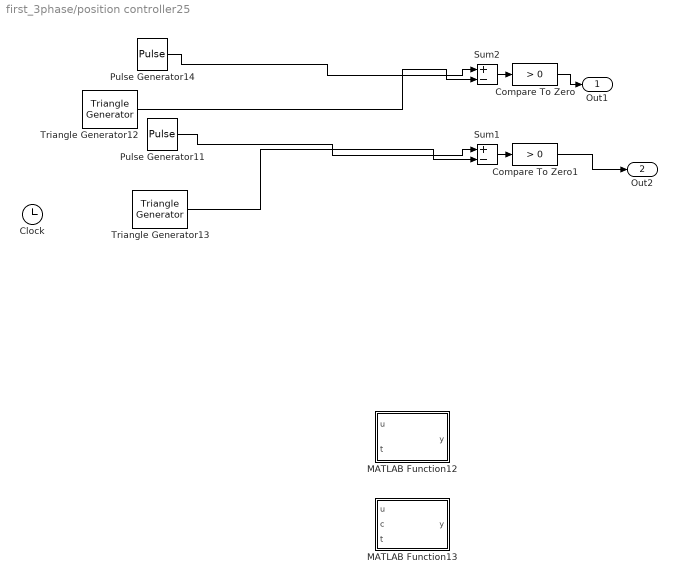
== system first_3phase/position controller25 ==
  Clock : Clock
  Compare To Zero : simulink/Logic and Bit Operations/Compare To Zero  relop=>  OutDataTypeStr=boolean  ZeroCross=off
  Compare To Zero1 : simulink/Logic and Bit Operations/Compare To Zero  relop=>  OutDataTypeStr=boolean  ZeroCross=off
  MATLAB Function12 : MATLAB Function  TreatAsAtomicUnit=on
  MATLAB Function13 : MATLAB Function  TreatAsAtomicUnit=on
  Pulse Generator11 : DiscretePulseGenerator  PulseType=Time based  Amplitude=0.9502  Period=0.02  PulseWidth=50  PhaseDelay=0.01+0.00666*2
  Pulse Generator14 : DiscretePulseGenerator  PulseType=Time based  Amplitude=0.9502  Period=0.966211111111111  PulseWidth=50  PhaseDelay=0.00666*2
  Sum1 : Sum  Inputs=+-  OutDataTypeStr=double
  Sum2 : Sum  Inputs=+-  OutDataTypeStr=double
  Triangle Generator12 : powerlib_meascontrol/Pulse & Signal Generators/Triangle Generator  Freq=50  Phase=90+120  Ts=0
  Triangle Generator13 : powerlib_meascontrol/Pulse & Signal Generators/Triangle Generator  Freq=50  Phase=90+180+120  Ts=0
  Out1 : Outport
  Out2 : Outport  Port=2
  wires:
  Compare To Zero/1 -> Out1/1
  Compare To Zero1/1 -> Out2/1
  Pulse Generator14/1 -> Sum2/1
  Triangle Generator12/1 -> Sum2/2
  Pulse Generator11/1 -> Sum1/1
  Triangle Generator13/1 -> Sum1/2
  Sum2/1 -> Compare To Zero/1
  Sum1/1 -> Compare To Zero1/1

== system first_3phase/position controller3 ==
  Compare To Zero : simulink/Logic and Bit Operations/Compare To Zero  relop=>  OutDataTypeStr=boolean  ZeroCross=off
  Compare To Zero1 : simulink/Logic and Bit Operations/Compare To Zero  relop=>  OutDataTypeStr=boolean  ZeroCross=off
  MATLAB Function14 : MATLAB Function  TreatAsAtomicUnit=on
  MATLAB Function15 : MATLAB Function  TreatAsAtomicUnit=on
  Pulse Generator5 : DiscretePulseGenerator  PulseType=Time based  Amplitude=0.332  Period=0.02  PulseWidth=50.001
  Pulse Generator6 : DiscretePulseGenerator  PulseType=Time based  Amplitude=0.332  Period=0.02  PulseWidth=50.001  PhaseDelay=0.01
  Sum1 : Sum  Inputs=+-  OutDataTypeStr=double
  Sum2 : Sum  Inputs=+-  OutDataTypeStr=double
  Triangle Generator4 : powerlib_meascontrol/Pulse & Signal Generators/Triangle Generator  Freq=50  Phase=90  Ts=0
  Triangle Generator5 : powerlib_meascontrol/Pulse & Signal Generators/Triangle Generator  Freq=50  Phase=90+180  Ts=0
  Out3 : Outport
  Out4 : Outport  Port=2
  wires:
  Compare To Zero/1 -> Out3/1
  Compare To Zero1/1 -> Out4/1
  Pulse Generator5/1 -> Sum2/2
  Triangle Generator4/1 -> Sum2/1
  Pulse Generator6/1 -> Sum1/2
  Triangle Generator5/1 -> Sum1/1
  Sum2/1 -> Compare To Zero/1
  Sum1/1 -> Compare To Zero1/1

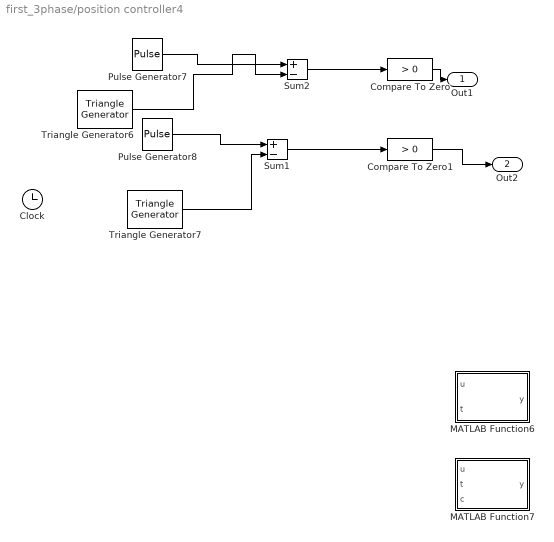
== system first_3phase/position controller4 ==
  Clock : Clock
  Compare To Zero : simulink/Logic and Bit Operations/Compare To Zero  relop=>  OutDataTypeStr=boolean  ZeroCross=off
  Compare To Zero1 : simulink/Logic and Bit Operations/Compare To Zero  relop=>  OutDataTypeStr=boolean  ZeroCross=off
  MATLAB Function6 : MATLAB Function  TreatAsAtomicUnit=on
  MATLAB Function7 : MATLAB Function  TreatAsAtomicUnit=on
  Pulse Generator7 : DiscretePulseGenerator  PulseType=Time based  Amplitude=0.666  Period=0.02  PulseWidth=50  PhaseDelay=0.00666
  Pulse Generator8 : DiscretePulseGenerator  PulseType=Time based  Amplitude=0.666  Period=0.02  PulseWidth=50  PhaseDelay=0.01+0.00666
  Sum1 : Sum  Inputs=+-  OutDataTypeStr=double
  Sum2 : Sum  Inputs=+-  OutDataTypeStr=double
  Triangle Generator6 : powerlib_meascontrol/Pulse & Signal Generators/Triangle Generator  Freq=50  Phase=90+240  Ts=0
  Triangle Generator7 : powerlib_meascontrol/Pulse & Signal Generators/Triangle Generator  Freq=50  Phase=90+180+240  Ts=0
  Out1 : Outport
  Out2 : Outport  Port=2
  wires:
  Compare To Zero/1 -> Out1/1
  Compare To Zero1/1 -> Out2/1
  Triangle Generator6/1 -> Sum2/2
  Pulse Generator8/1 -> Sum1/1
  Pulse Generator7/1 -> Sum2/1
  Triangle Generator7/1 -> Sum1/2
  Sum2/1 -> Compare To Zero/1
  Sum1/1 -> Compare To Zero1/1

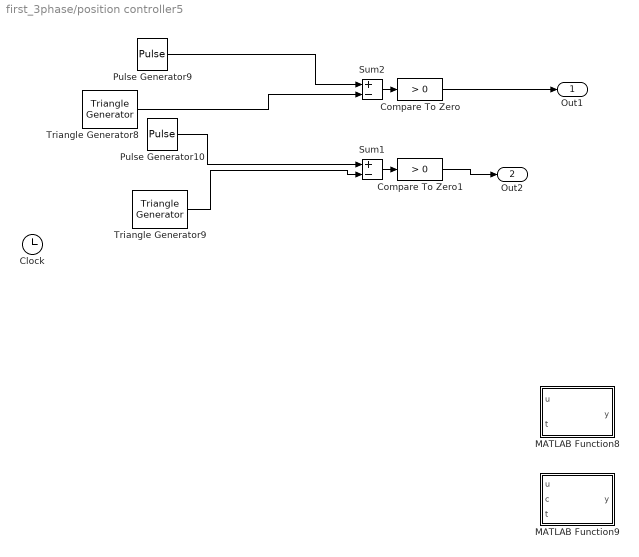
== system first_3phase/position controller5 ==
  Clock : Clock
  Compare To Zero : simulink/Logic and Bit Operations/Compare To Zero  relop=>  OutDataTypeStr=boolean  ZeroCross=off
  Compare To Zero1 : simulink/Logic and Bit Operations/Compare To Zero  relop=>  OutDataTypeStr=boolean  ZeroCross=off
  MATLAB Function8 : MATLAB Function  TreatAsAtomicUnit=on
  MATLAB Function9 : MATLAB Function  TreatAsAtomicUnit=on
  Pulse Generator10 : DiscretePulseGenerator  PulseType=Time based  Amplitude=0.333  Period=0.02  PulseWidth=50  PhaseDelay=0.01+0.00666
  Pulse Generator9 : DiscretePulseGenerator  PulseType=Time based  Amplitude=0.333  Period=0.02  PulseWidth=50  PhaseDelay=0.00666
  Sum1 : Sum  Inputs=+-  OutDataTypeStr=double
  Sum2 : Sum  Inputs=+-  OutDataTypeStr=double
  Triangle Generator8 : powerlib_meascontrol/Pulse & Signal Generators/Triangle Generator  Freq=50  Phase=90+240  Ts=0
  Triangle Generator9 : powerlib_meascontrol/Pulse & Signal Generators/Triangle Generator  Freq=50  Phase=90+180+240  Ts=0
  Out1 : Outport
  Out2 : Outport  Port=2
  wires:
  Compare To Zero/1 -> Out1/1
  Triangle Generator8/1 -> Sum2/2
  Compare To Zero1/1 -> Out2/1
  Pulse Generator10/1 -> Sum1/1
  Triangle Generator9/1 -> Sum1/2
  Sum2/1 -> Compare To Zero/1
  Sum1/1 -> Compare To Zero1/1
  Pulse Generator9/1 -> Sum2/1

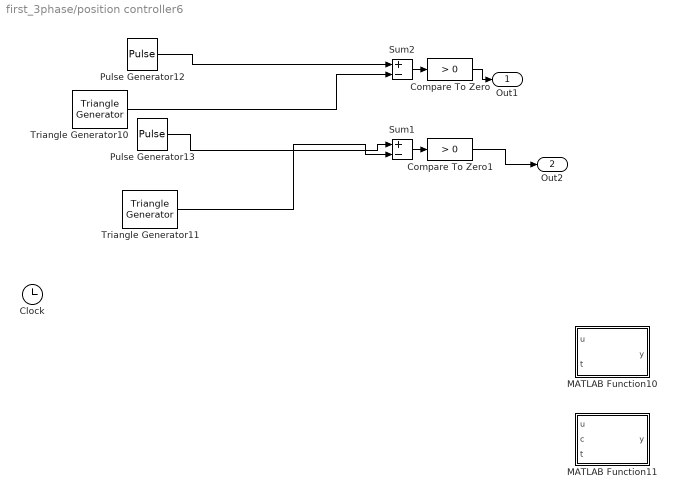
== system first_3phase/position controller6 ==
  Clock : Clock
  Compare To Zero : simulink/Logic and Bit Operations/Compare To Zero  relop=>  OutDataTypeStr=boolean  ZeroCross=off
  Compare To Zero1 : simulink/Logic and Bit Operations/Compare To Zero  relop=>  OutDataTypeStr=boolean  ZeroCross=off
  MATLAB Function10 : MATLAB Function  TreatAsAtomicUnit=on
  MATLAB Function11 : MATLAB Function  TreatAsAtomicUnit=on
  Pulse Generator12 : DiscretePulseGenerator  PulseType=Time based  Amplitude=0.666  Period=0.02  PulseWidth=50  PhaseDelay=0.00666*2
  Pulse Generator13 : DiscretePulseGenerator  PulseType=Time based  Amplitude=0.666  Period=0.02  PulseWidth=50  PhaseDelay=0.01+0.00666*2
  Sum1 : Sum  Inputs=+-  OutDataTypeStr=double
  Sum2 : Sum  Inputs=+-  OutDataTypeStr=double
  Triangle Generator10 : powerlib_meascontrol/Pulse & Signal Generators/Triangle Generator  Freq=50  Phase=90+120  Ts=0
  Triangle Generator11 : powerlib_meascontrol/Pulse & Signal Generators/Triangle Generator  Freq=50  Phase=90+180+120  Ts=0
  Out1 : Outport
  Out2 : Outport  Port=2
  wires:
  Compare To Zero/1 -> Out1/1
  Compare To Zero1/1 -> Out2/1
  Triangle Generator10/1 -> Sum2/2
  Pulse Generator13/1 -> Sum1/1
  Triangle Generator11/1 -> Sum1/2
  Pulse Generator12/1 -> Sum2/1
  Sum2/1 -> Compare To Zero/1
  Sum1/1 -> Compare To Zero1/1

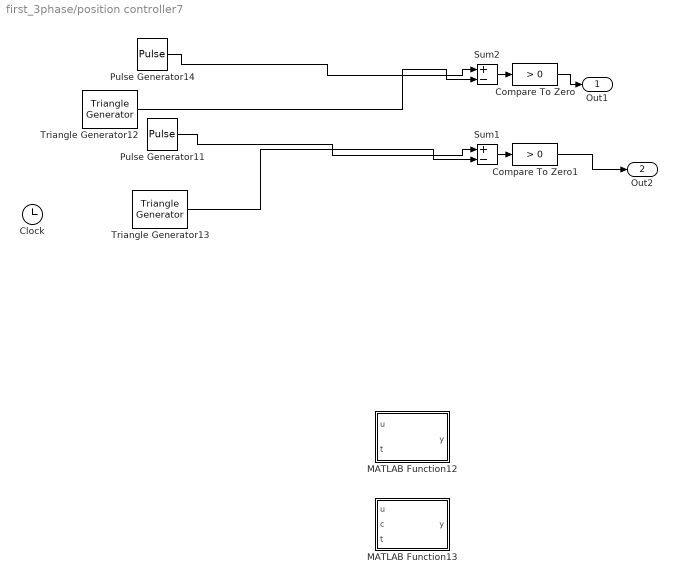
== system first_3phase/position controller7 ==
  Clock : Clock
  Compare To Zero : simulink/Logic and Bit Operations/Compare To Zero  relop=>  OutDataTypeStr=boolean  ZeroCross=off
  Compare To Zero1 : simulink/Logic and Bit Operations/Compare To Zero  relop=>  OutDataTypeStr=boolean  ZeroCross=off
  MATLAB Function12 : MATLAB Function  TreatAsAtomicUnit=on
  MATLAB Function13 : MATLAB Function  TreatAsAtomicUnit=on
  Pulse Generator11 : DiscretePulseGenerator  PulseType=Time based  Amplitude=0.333  Period=0.02  PulseWidth=50  PhaseDelay=0.01+0.00666*2
  Pulse Generator14 : DiscretePulseGenerator  PulseType=Time based  Amplitude=0.333  Period=0.02  PulseWidth=50  PhaseDelay=0.00666*2
  Sum1 : Sum  Inputs=+-  OutDataTypeStr=double
  Sum2 : Sum  Inputs=+-  OutDataTypeStr=double
  Triangle Generator12 : powerlib_meascontrol/Pulse & Signal Generators/Triangle Generator  Freq=50  Phase=90+120  Ts=0
  Triangle Generator13 : powerlib_meascontrol/Pulse & Signal Generators/Triangle Generator  Freq=50  Phase=90+180+120  Ts=0
  Out1 : Outport
  Out2 : Outport  Port=2
  wires:
  Compare To Zero/1 -> Out1/1
  Compare To Zero1/1 -> Out2/1
  Pulse Generator14/1 -> Sum2/1
  Triangle Generator12/1 -> Sum2/2
  Pulse Generator11/1 -> Sum1/1
  Triangle Generator13/1 -> Sum1/2
  Sum2/1 -> Compare To Zero/1
  Sum1/1 -> Compare To Zero1/1

== system first_3phase/position controller8 ==
  Pulse Generator : DiscretePulseGenerator  PulseType=Time based  Period=0.02  PulseWidth=50
  Pulse Generator4 : DiscretePulseGenerator  PulseType=Time based  Period=0.02  PulseWidth=50  PhaseDelay=0.01
  Triangle Generator : powerlib_meascontrol/Pulse & Signal Generators/Triangle Generator  Freq=50  Phase=90  Ts=0
  Triangle Generator3 : powerlib_meascontrol/Pulse & Signal Generators/Triangle Generator  Freq=50  Phase=90+180  Ts=0
  Out1 : Outport
  Out2 : Outport  Port=2
  wires:
  Pulse Generator/1 -> Out1/1
  Triangle Generator/1 -> ?
  Triangle Generator3/1 -> ?
  Pulse Generator4/1 -> Out2/1

== system first_3phase/position controller9 ==
  Pulse Generator5 : DiscretePulseGenerator  PulseType=Time based  Period=0.02  PulseWidth=50
  Pulse Generator6 : DiscretePulseGenerator  PulseType=Time based  Period=0.02  PulseWidth=50  PhaseDelay=0.01
  Triangle Generator4 : powerlib_meascontrol/Pulse & Signal Generators/Triangle Generator  Freq=50  Phase=90  Ts=0
  Triangle Generator5 : powerlib_meascontrol/Pulse & Signal Generators/Triangle Generator  Freq=50  Phase=90+180  Ts=0
  Out1 : Outport
  Out2 : Outport  Port=2
  wires:
  Pulse Generator5/1 -> Out1/1
  Triangle Generator4/1 -> ?
  Pulse Generator6/1 -> Out2/1

== matlab function first_3phase/position controller3/MATLAB Function14 ==
  data: u input; y output; t input
function y = fcn(u,t)
%#codegen
if t>u
    y = 1;
else
    y = 0;
end
end

== matlab function first_3phase/position controller17/MATLAB Function ==
  data: u input; y output; t input
function y = fcn(u,t)
%#codegen
if t>u
    y = 1;
else
    y = 0;
end
end

== matlab function first_3phase/position controller4/MATLAB Function6 ==
  data: u input; y output; t input
function y = fcn(u,t)
%#codegen
if t>u
    y = 1;
else
    y = 0;
end
end

== matlab function first_3phase/position controller17/MATLAB Function3 ==
  data: u input; y output; t input
function y = fcn(u,t)
%#codegen
if t>u
    y = 1;
else
    y = 0;
end
end

== matlab function first_3phase/position controller2/MATLAB Function1 ==
  data: u input; y output; t input
function y = fcn(u,t)
%#codegen
if t>u
    y = 1;
else
    y = 0;
end
end

== matlab function first_3phase/position controller2/MATLAB Function2 ==
  data: u input; y output; t input
function y = fcn(u,t)
%#codegen
if t>u
    y = 1;
else
    y = 0;
end
end

== matlab function first_3phase/position controller5/MATLAB Function8 ==
  data: u input; y output; t input
function y = fcn(u,t)
%#codegen
if t>u
    y = 1;
else
    y = 0;
end
end

== matlab function first_3phase/position controller5/MATLAB Function9 ==
  data: u input; c input; y output; t input
function y = fcn(u,c,t)
%#codegen
if t>u
    y = 1;
else
    y = 0;
end
if c <0.02
    y = 0;
end

== matlab function first_3phase/position controller7/MATLAB Function12 ==
  data: u input; y output; t input
function y = fcn(u,t)
%#codegen
if t>u
    y = 1;
else
    y = 0;
end
end

== matlab function first_3phase/position controller7/MATLAB Function13 ==
  data: u input; c input; y output; t input
function y = fcn(u,c,t)
%#codegen
if t>u
    y = 1;
else
    y = 0;
end
if c<0.02
    y = 0;
end

== matlab function first_3phase/position controller22/MATLAB Function6 ==
  data: u input; y output; t input
function y = fcn(u,t)
%#codegen
if t>u
    y = 1;
else
    y = 0;
end
end

== matlab function first_3phase/position controller22/MATLAB Function7 ==
  data: u input; y output; t input; c input
function y = fcn(u,t,c)
%#codegen
if t>u
    y = 1;
else
    y = 0;
end
if c<0.02
    y =0;
end

== matlab function first_3phase/position controller11/MATLAB Function8 ==
  data: u input; y output; t input
function y = fcn(u,t)
%#codegen
if t>u
    y = 1;
else
    y = 0;
end
end

== matlab function first_3phase/position controller11/MATLAB Function9 ==
  data: u input; c input; y output; t input
function y = fcn(u,c,t)
%#codegen
if t>u
    y = 1;
else
    y = 0;
end
if c <0.02
    y = 0;
end

== matlab function first_3phase/position controller4/MATLAB Function7 ==
  data: u input; y output; t input; c input
function y = fcn(u,t,c)
%#codegen
if t>u
    y = 1;
else
    y = 0;
end
if c<0.02
    y =0;
end

== matlab function first_3phase/position controller3/MATLAB Function15 ==
  data: u input; y output; t input
function y = fcn(u,t)
%#codegen
if t>u
    y = 1;
else
    y = 0;
end
end

== matlab function first_3phase/position controller/MATLAB Function ==
  data: u input; y output; t input
function y = fcn(u,t)
%#codegen
if t>u
    y = 1;
else
    y = 0;
end
end

== matlab function first_3phase/position controller/MATLAB Function3 ==
  data: u input; y output; t input
function y = fcn(u,t)
%#codegen
if t>u
    y = 1;
else
    y = 0;
end
end

== matlab function first_3phase/position controller23/MATLAB Function8 ==
  data: u input; y output; t input
function y = fcn(u,t)
%#codegen
if t>u
    y = 1;
else
    y = 0;
end
end

== matlab function first_3phase/position controller23/MATLAB Function9 ==
  data: u input; c input; y output; t input
function y = fcn(u,c,t)
%#codegen
if t>u
    y = 1;
else
    y = 0;
end
if c <0.02
    y = 0;
end

== matlab function first_3phase/position controller6/MATLAB Function10 ==
  data: u input; y output; t input
function y = fcn(u,t)
%#codegen
if t>u
    y = 1;
else
    y = 0;
end
end

== matlab function first_3phase/position controller6/MATLAB Function11 ==
  data: u input; c input; y output; t input
function y = fcn(u,c,t)
%#codegen
if t>u
    y = 1;
else
    y = 0;
end
if c<0.02
    y = 0;
end

== matlab function first_3phase/position controller24/MATLAB Function10 ==
  data: u input; y output; t input
function y = fcn(u,t)
%#codegen
if t>u
    y = 1;
else
    y = 0;
end
end

== matlab function first_3phase/position controller24/MATLAB Function11 ==
  data: u input; c input; y output; t input
function y = fcn(u,c,t)
%#codegen
if t>u
    y = 1;
else
    y = 0;
end
if c<0.02
    y = 0;
end

== matlab function first_3phase/position controller25/MATLAB Function12 ==
  data: u input; y output; t input
function y = fcn(u,t)
%#codegen
if t>u
    y = 1;
else
    y = 0;
end
end

== matlab function first_3phase/position controller25/MATLAB Function13 ==
  data: u input; c input; y output; t input
function y = fcn(u,c,t)
%#codegen
if t>u
    y = 1;
else
    y = 0;
end
if c<0.02
    y = 0;
end
